simulink model "PD_Controller"  (R2023b)
settings: Solver=VariableStepAuto  StartTime=0.0  StopTime=20  RelTol=1e-3
settings Model: Creator=patel  LastModifiedBy=patel

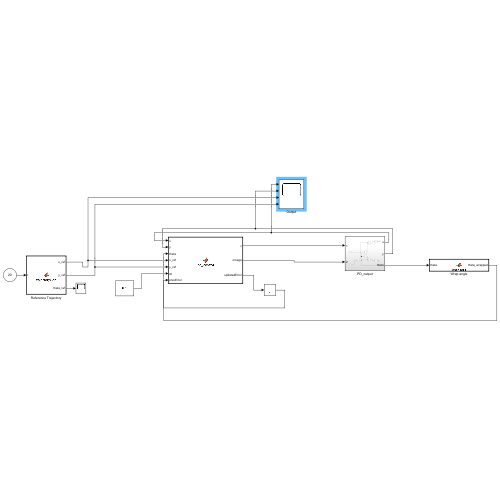
[thumbnail: Simulink's stored preview of the top-level diagram]
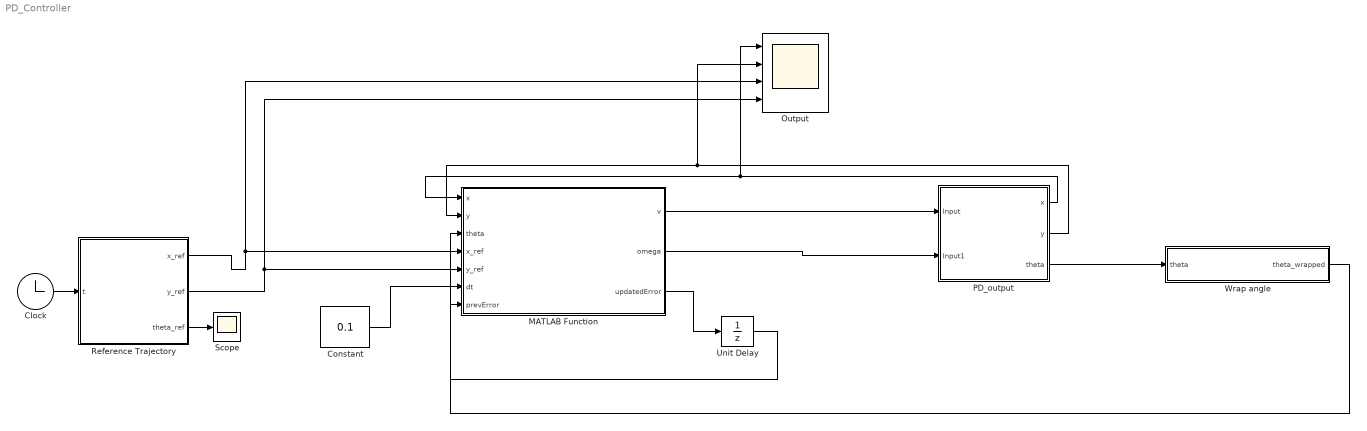
== system PD_Controller ==
  Clock : Clock
      settings: Decimation=20
  Constant : Constant  Value=0.1
  MATLAB Function : MATLAB Function  TreatAsAtomicUnit=on
  Output : Scope  NumInputPorts=4
  PD_output : Subsystem
  Reference Trajectory : MATLAB Function  TreatAsAtomicUnit=on
  Scope : Scope
  Unit Delay : UnitDelay  SampleTime=-1  HasFrameUpgradeWarning=on
  Wrap angle : MATLAB Function  TreatAsAtomicUnit=on
  wires:
  PD_output/1(x) -> MATLAB Function/1(x), Output/1
  Reference Trajectory/2(y_ref) -> MATLAB Function/5(y_ref), Output/4
  Clock/1 -> Reference Trajectory/1(t)
  Reference Trajectory/3(theta_ref) -> Scope/1
  Reference Trajectory/1(x_ref) -> MATLAB Function/4(x_ref), Output/3
  PD_output/2(y) -> MATLAB Function/2(y), Output/2
  Wrap angle/1(theta_wrapped) -> MATLAB Function/3(theta)
  PD_output/3(theta) -> Wrap angle/1(theta)
  Constant/1 -> MATLAB Function/6(dt)
  MATLAB Function/3(updatedError) -> Unit Delay/1
  Unit Delay/1 -> MATLAB Function/7(prevError)
  MATLAB Function/1(v) -> PD_output/1(Input)
  MATLAB Function/2(omega) -> PD_output/2(Input1)

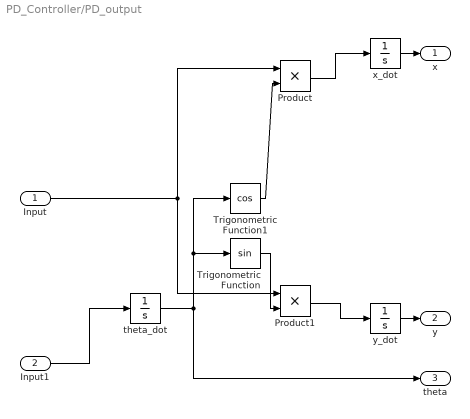
== system PD_Controller/PD_output ==
  Input : Inport
  Input1 : Inport  Port=2
  Product : Product
  Product1 : Product
  Trigonometric Function : Trigonometry
  Trigonometric Function1 : Trigonometry  Operator=cos
  theta_dot : Integrator
  x_dot : Integrator
  y_dot : Integrator
  x : Outport
  y : Outport  Port=2
  theta : Outport  Port=3
  wires:
  theta_dot/1 -> theta/1, Trigonometric Function1/1, Trigonometric Function/1
  Product/1 -> x_dot/1
  Input1/1 -> theta_dot/1
  Trigonometric Function1/1 -> Product/2
  Input/1 -> Product1/1, Product/1
  Trigonometric Function/1 -> Product1/2
  Product1/1 -> y_dot/1
  x_dot/1 -> x/1
  y_dot/1 -> y/1

== matlab function PD_Controller/Reference Trajectory ==
  data: t input; x_ref output; y_ref output; theta_ref output
function [x_ref, y_ref, theta_ref] = trajectoryGen(t)
    radius = 5;
    omega_ref = 0.2;
    x_ref = radius * cos(omega_ref * t);
    y_ref = radius * sin(omega_ref * t);
    theta_ref = omega_ref * t + pi/2;
end

== matlab function PD_Controller/Wrap angle ==
  data: theta input; theta_wrapped output
function theta_wrapped = wrapToPi(theta)
    theta_wrapped = mod(theta + pi, 2*pi) - pi;
end

== matlab function PD_Controller/MATLAB Function ==
  data: x input; v output; y input; theta input; x_ref input; y_ref input; dt input; prevError input; omega output; updatedError output

function [v, omega, updatedError] = pd_control(x, y, theta, x_ref, y_ref, dt, prevError)
%#codegen
robotState = [x; y; theta];
targetPoint = [x_ref; y_ref];
[v, omega, updatedError] = PD_Controller(robotState, targetPoint, dt, prevError);

    function [v, omega, updatedPrevAngleError] = PD_Controller(robotState, targetPoint, dt, prevAngleError)
    x = robotState(1); y = robotState(2); theta = robotState(3);
    x_target = targetPoint(1); y_target = targetPoint(2);

    dx = x_target - x;
    dy = y_target - y;
    dist_to_target = sqrt(dx^2 + dy^2);

    angle_to_target = atan2(dy, dx);
    angle_error = atan2(sin(angle_to_target - theta), cos(angle_to_target - theta));
    angle_error_deriv = (angle_error - prevAngleError) / dt;
    updatedPrevAngleError = angle_error;

    % PD Gains
    kp_v = 1.5;
    kp_omega = 2.0;
    kd_omega = 1.0;

    v = min(max(kp_v * dist_to_target, 0.2), 5.0);
    omega = min(max(kp_omega * angle_error + kd_omega * angle_error_deriv, -pi), pi);
end

end
